simulink model "eVTOL_System"  (R2024b)
settings: Solver=FixedStepAuto  StartTime=0.0  StopTime=inf  RelTol=1e-3
undefined symbols (not defined in the file): airspeed, Battery, BCE12, BCE_Set_init, BMS_Controller_State, C, Cell10_P, Cell11_P, Cell12_P, Cell13_P, Cell14_P, Cell15_P, Cell16_P, Cell17_P, Cell18_P, Cell19_P, Cell1_N, Cell1_P, Cell20_P, Cell21_P, Cell22_P, Cell23_P, Cell24_P, Cell2_P, Cell3_P, Cell4_P, Cell5_P, Cell6_P, Cell7_P, Cell8_P, Cell9_P, Charging_State, CityMission, control, controlParams, ControlSampleTime, CriticalTiltAngle, currentFactor, CV_Gain, ddx, ddy, ddz, Device_01, Device_02, DiscIntNeverNeededParam, dx, dy, dz, Earth, env, F, F28379D_ADC_MaxCount, F28379D_ADC_Vmax, FixedWingMission, flightState, Foc_Ki_IxTcpu, Foc_Ki_S, Foc_Kp_I, Foc_Kp_S, fractalcoef ... (+68)
libraries: fl_lib x1115, nesl_utility x617, slrealtimeethercatlib x217, simulink x130, canmsglib x101, speedgoatlib_IO611_obsolete x91, slpidlib x49, mcbcontrolslib x44, slrealtimeutilitieslib x35, speedgoatlib_hdlCoder_IO3xx x31, dspstat3 x24, mcbpositiondecoderlib x12
(part 8 of 31)

== system eVTOL_System/Motor Drive/Controller/Controller_MIL/F28379D Firmware ==
  Ia_ADC : Inport
  Ib_ADC : Inport  Port=2
  IaOffset : Inport  Port=3
  IbOffset : Inport  Port=4
  QEP_Position_Count : Inport  Port=5
  QEP_Index_Latch : Inport  Port=6
  SpdCmdRPM : Inport  Port=7
  Kp_S : Inport  Port=8
  Ki_S : Inport  Port=9
  EnClosedLoop : Inport  Port=10
  EnablePWM : Inport  Port=11
  Kp_i : Inport  Port=12
  Ki_ixTcpu : Inport  Port=13
  Controller Algorithm : Subsystem
  Phase_Current_Rescaling : Subsystem
  Speed Conditioning : Subsystem
  ModWave : Outport
  PWM_Enable : Outport  Port=2
  Fbk_CAN : Outport  Port=3
  wires:
  SpdCmdRPM/1 -> Speed Conditioning/1(Spd[rpm])
  Ia_ADC/1 -> Phase_Current_Rescaling/1(Ia_ADC)
  IaOffset/1 -> Phase_Current_Rescaling/3(IaOffset)
  IbOffset/1 -> Phase_Current_Rescaling/4(IbOffset)
  QEP_Position_Count/1 -> Controller Algorithm/2(QEP_Position_Count)
  Controller Algorithm/1(ModWave) -> ModWave/1
  Phase_Current_Rescaling/1(Iab_meas_PU) -> Controller Algorithm/1(Ia_PU)  "Iab_fb_PU"
  Kp_S/1 -> Controller Algorithm/5(Kp_S)
  Controller Algorithm/2(PWM_Enable) -> PWM_Enable/1
  Ki_S/1 -> Controller Algorithm/6(Ki_S)
  QEP_Index_Latch/1 -> Controller Algorithm/3(QEP_Index_Latch)
  Ib_ADC/1 -> Phase_Current_Rescaling/2(Ib_ADC)
  EnClosedLoop/1 -> Controller Algorithm/7(EnClosedLoop)
  EnablePWM/1 -> Controller Algorithm/8(EnablePWM)
  Speed Conditioning/1(Spd[PU]) -> Controller Algorithm/4(SpdCmd)
  Controller Algorithm/3(fbk_CAN) -> Fbk_CAN/1
  Kp_i/1 -> Controller Algorithm/9(Kp_i)
  Ki_ixTcpu/1 -> Controller Algorithm/10(Ki_ixTcpu)

== system eVTOL_System/Motor Drive/Controller/Controller_MIL/IO334 DAC ==
  Iab : Inport
  Add : Sum
  Constant : Constant  Value=IO334_iDAC_bias
  Gain : Gain  Gain=IO334_iDAC_gain
  Gain1 : Gain  Gain=2.5/(2^15)
  IO334_DAC_embedded_GAIN : Gain  Gain=2^15/10
  Saturation : Saturate  UpperLimit=IO334_DAC_Vmax  LowerLimit=-IO334_DAC_Vmax
  Iab_IO334DAC : Outport
  wires:
  Iab/1 -> Gain/1
  Gain/1 -> Add/1
  Add/1 -> IO334_DAC_embedded_GAIN/1
  Constant/1 -> Add/2
  IO334_DAC_embedded_GAIN/1 -> Gain1/1
  Gain1/1 -> Saturation/1
  Saturation/1 -> Iab_IO334DAC/1

== system eVTOL_System/Motor Drive/Controller1/Controller_MIL/F28379D ADC ==
  Iab_IO334V : Inport
  Add Constant : Bias  Bias=Ia_offset  SaturateOnIntegerOverflow=off
  Add Constant1 : Bias  Bias=Ib_offset  SaturateOnIntegerOverflow=off
  Demux : Demux  Outputs=2
  Gain : Gain  Gain=2^12/F28379D_ADC_Vmax
  Ia_ADC : Outport
  Ib_ADC : Outport  Port=2
  wires:
  Iab_IO334V/1 -> Gain/1
  Gain/1 -> Demux/1
  Demux/1 -> Add Constant/1
  Demux/2 -> Add Constant1/1
  Add Constant/1 -> Ia_ADC/1
  Add Constant1/1 -> Ib_ADC/1

== system eVTOL_System/Motor Drive/Controller1/Controller_MIL/F28379D Firmware ==
  Ia_ADC : Inport
  Ib_ADC : Inport  Port=2
  IaOffset : Inport  Port=3
  IbOffset : Inport  Port=4
  QEP_Position_Count : Inport  Port=5
  QEP_Index_Latch : Inport  Port=6
  SpdCmdRPM : Inport  Port=7
  Kp_S : Inport  Port=8
  Ki_S : Inport  Port=9
  EnClosedLoop : Inport  Port=10
  EnablePWM : Inport  Port=11
  Kp_i : Inport  Port=12
  Ki_ixTcpu : Inport  Port=13
  Controller Algorithm : Subsystem
  Phase_Current_Rescaling : Subsystem
  Speed Conditioning : Subsystem
  ModWave : Outport
  PWM_Enable : Outport  Port=2
  Fbk_CAN : Outport  Port=3
  wires:
  SpdCmdRPM/1 -> Speed Conditioning/1(Spd[rpm])
  Ia_ADC/1 -> Phase_Current_Rescaling/1(Ia_ADC)
  IaOffset/1 -> Phase_Current_Rescaling/3(IaOffset)
  IbOffset/1 -> Phase_Current_Rescaling/4(IbOffset)
  QEP_Position_Count/1 -> Controller Algorithm/2(QEP_Position_Count)
  Controller Algorithm/1(ModWave) -> ModWave/1
  Phase_Current_Rescaling/1(Iab_meas_PU) -> Controller Algorithm/1(Ia_PU)  "Iab_fb_PU"
  Kp_S/1 -> Controller Algorithm/5(Kp_S)
  Controller Algorithm/2(PWM_Enable) -> PWM_Enable/1
  Ki_S/1 -> Controller Algorithm/6(Ki_S)
  QEP_Index_Latch/1 -> Controller Algorithm/3(QEP_Index_Latch)
  Ib_ADC/1 -> Phase_Current_Rescaling/2(Ib_ADC)
  EnClosedLoop/1 -> Controller Algorithm/7(EnClosedLoop)
  EnablePWM/1 -> Controller Algorithm/8(EnablePWM)
  Speed Conditioning/1(Spd[PU]) -> Controller Algorithm/4(SpdCmd)
  Controller Algorithm/3(fbk_CAN) -> Fbk_CAN/1
  Kp_i/1 -> Controller Algorithm/9(Kp_i)
  Ki_ixTcpu/1 -> Controller Algorithm/10(Ki_ixTcpu)

== system eVTOL_System/Motor Drive/Controller1/Controller_MIL/IO334 DAC ==
  Iab : Inport
  Add : Sum
  Constant : Constant  Value=IO334_iDAC_bias
  Gain : Gain  Gain=IO334_iDAC_gain
  Gain1 : Gain  Gain=2.5/(2^15)
  IO334_DAC_embedded_GAIN : Gain  Gain=2^15/10
  Saturation : Saturate  UpperLimit=IO334_DAC_Vmax  LowerLimit=-IO334_DAC_Vmax
  Iab_IO334DAC : Outport
  wires:
  Iab/1 -> Gain/1
  Gain/1 -> Add/1
  Add/1 -> IO334_DAC_embedded_GAIN/1
  Constant/1 -> Add/2
  IO334_DAC_embedded_GAIN/1 -> Gain1/1
  Gain1/1 -> Saturation/1
  Saturation/1 -> Iab_IO334DAC/1

== system eVTOL_System/Motor Drive/Controller2/Controller_MIL/F28379D ADC ==
  Iab_IO334V : Inport
  Add Constant : Bias  Bias=Ia_offset  SaturateOnIntegerOverflow=off
  Add Constant1 : Bias  Bias=Ib_offset  SaturateOnIntegerOverflow=off
  Demux : Demux  Outputs=2
  Gain : Gain  Gain=2^12/F28379D_ADC_Vmax
  Ia_ADC : Outport
  Ib_ADC : Outport  Port=2
  wires:
  Iab_IO334V/1 -> Gain/1
  Gain/1 -> Demux/1
  Demux/1 -> Add Constant/1
  Demux/2 -> Add Constant1/1
  Add Constant/1 -> Ia_ADC/1
  Add Constant1/1 -> Ib_ADC/1

== system eVTOL_System/Motor Drive/Controller2/Controller_MIL/F28379D Firmware ==
  Ia_ADC : Inport
  Ib_ADC : Inport  Port=2
  IaOffset : Inport  Port=3
  IbOffset : Inport  Port=4
  QEP_Position_Count : Inport  Port=5
  QEP_Index_Latch : Inport  Port=6
  SpdCmdRPM : Inport  Port=7
  Kp_S : Inport  Port=8
  Ki_S : Inport  Port=9
  EnClosedLoop : Inport  Port=10
  EnablePWM : Inport  Port=11
  Kp_i : Inport  Port=12
  Ki_ixTcpu : Inport  Port=13
  Controller Algorithm : Subsystem
  Phase_Current_Rescaling : Subsystem
  Speed Conditioning : Subsystem
  ModWave : Outport
  PWM_Enable : Outport  Port=2
  Fbk_CAN : Outport  Port=3
  wires:
  SpdCmdRPM/1 -> Speed Conditioning/1(Spd[rpm])
  Ia_ADC/1 -> Phase_Current_Rescaling/1(Ia_ADC)
  IaOffset/1 -> Phase_Current_Rescaling/3(IaOffset)
  IbOffset/1 -> Phase_Current_Rescaling/4(IbOffset)
  QEP_Position_Count/1 -> Controller Algorithm/2(QEP_Position_Count)
  Controller Algorithm/1(ModWave) -> ModWave/1
  Phase_Current_Rescaling/1(Iab_meas_PU) -> Controller Algorithm/1(Ia_PU)  "Iab_fb_PU"
  Kp_S/1 -> Controller Algorithm/5(Kp_S)
  Controller Algorithm/2(PWM_Enable) -> PWM_Enable/1
  Ki_S/1 -> Controller Algorithm/6(Ki_S)
  QEP_Index_Latch/1 -> Controller Algorithm/3(QEP_Index_Latch)
  Ib_ADC/1 -> Phase_Current_Rescaling/2(Ib_ADC)
  EnClosedLoop/1 -> Controller Algorithm/7(EnClosedLoop)
  EnablePWM/1 -> Controller Algorithm/8(EnablePWM)
  Speed Conditioning/1(Spd[PU]) -> Controller Algorithm/4(SpdCmd)
  Controller Algorithm/3(fbk_CAN) -> Fbk_CAN/1
  Kp_i/1 -> Controller Algorithm/9(Kp_i)
  Ki_ixTcpu/1 -> Controller Algorithm/10(Ki_ixTcpu)

== system eVTOL_System/Motor Drive/Controller2/Controller_MIL/IO334 DAC ==
  Iab : Inport
  Add : Sum
  Constant : Constant  Value=IO334_iDAC_bias
  Gain : Gain  Gain=IO334_iDAC_gain
  Gain1 : Gain  Gain=2.5/(2^15)
  IO334_DAC_embedded_GAIN : Gain  Gain=2^15/10
  Saturation : Saturate  UpperLimit=IO334_DAC_Vmax  LowerLimit=-IO334_DAC_Vmax
  Iab_IO334DAC : Outport
  wires:
  Iab/1 -> Gain/1
  Gain/1 -> Add/1
  Add/1 -> IO334_DAC_embedded_GAIN/1
  Constant/1 -> Add/2
  IO334_DAC_embedded_GAIN/1 -> Gain1/1
  Gain1/1 -> Saturation/1
  Saturation/1 -> Iab_IO334DAC/1

== system eVTOL_System/Motor Drive/Controller3/Controller_MIL/F28379D ADC ==
  Iab_IO334V : Inport
  Add Constant : Bias  Bias=Ia_offset  SaturateOnIntegerOverflow=off
  Add Constant1 : Bias  Bias=Ib_offset  SaturateOnIntegerOverflow=off
  Demux : Demux  Outputs=2
  Gain : Gain  Gain=2^12/F28379D_ADC_Vmax
  Ia_ADC : Outport
  Ib_ADC : Outport  Port=2
  wires:
  Iab_IO334V/1 -> Gain/1
  Gain/1 -> Demux/1
  Demux/1 -> Add Constant/1
  Demux/2 -> Add Constant1/1
  Add Constant/1 -> Ia_ADC/1
  Add Constant1/1 -> Ib_ADC/1

== system eVTOL_System/Motor Drive/Controller3/Controller_MIL/F28379D Firmware ==
  Ia_ADC : Inport
  Ib_ADC : Inport  Port=2
  IaOffset : Inport  Port=3
  IbOffset : Inport  Port=4
  QEP_Position_Count : Inport  Port=5
  QEP_Index_Latch : Inport  Port=6
  SpdCmdRPM : Inport  Port=7
  Kp_S : Inport  Port=8
  Ki_S : Inport  Port=9
  EnClosedLoop : Inport  Port=10
  EnablePWM : Inport  Port=11
  Kp_i : Inport  Port=12
  Ki_ixTcpu : Inport  Port=13
  Controller Algorithm : Subsystem
  Phase_Current_Rescaling : Subsystem
  Speed Conditioning : Subsystem
  ModWave : Outport
  PWM_Enable : Outport  Port=2
  Fbk_CAN : Outport  Port=3
  wires:
  SpdCmdRPM/1 -> Speed Conditioning/1(Spd[rpm])
  Ia_ADC/1 -> Phase_Current_Rescaling/1(Ia_ADC)
  IaOffset/1 -> Phase_Current_Rescaling/3(IaOffset)
  IbOffset/1 -> Phase_Current_Rescaling/4(IbOffset)
  QEP_Position_Count/1 -> Controller Algorithm/2(QEP_Position_Count)
  Controller Algorithm/1(ModWave) -> ModWave/1
  Phase_Current_Rescaling/1(Iab_meas_PU) -> Controller Algorithm/1(Ia_PU)  "Iab_fb_PU"
  Kp_S/1 -> Controller Algorithm/5(Kp_S)
  Controller Algorithm/2(PWM_Enable) -> PWM_Enable/1
  Ki_S/1 -> Controller Algorithm/6(Ki_S)
  QEP_Index_Latch/1 -> Controller Algorithm/3(QEP_Index_Latch)
  Ib_ADC/1 -> Phase_Current_Rescaling/2(Ib_ADC)
  EnClosedLoop/1 -> Controller Algorithm/7(EnClosedLoop)
  EnablePWM/1 -> Controller Algorithm/8(EnablePWM)
  Speed Conditioning/1(Spd[PU]) -> Controller Algorithm/4(SpdCmd)
  Controller Algorithm/3(fbk_CAN) -> Fbk_CAN/1
  Kp_i/1 -> Controller Algorithm/9(Kp_i)
  Ki_ixTcpu/1 -> Controller Algorithm/10(Ki_ixTcpu)

== system eVTOL_System/Motor Drive/Controller3/Controller_MIL/IO334 DAC ==
  Iab : Inport
  Add : Sum
  Constant : Constant  Value=IO334_iDAC_bias
  Gain : Gain  Gain=IO334_iDAC_gain
  Gain1 : Gain  Gain=2.5/(2^15)
  IO334_DAC_embedded_GAIN : Gain  Gain=2^15/10
  Saturation : Saturate  UpperLimit=IO334_DAC_Vmax  LowerLimit=-IO334_DAC_Vmax
  Iab_IO334DAC : Outport
  wires:
  Iab/1 -> Gain/1
  Gain/1 -> Add/1
  Add/1 -> IO334_DAC_embedded_GAIN/1
  Constant/1 -> Add/2
  IO334_DAC_embedded_GAIN/1 -> Gain1/1
  Gain1/1 -> Saturation/1
  Saturation/1 -> Iab_IO334DAC/1

== system eVTOL_System/Motor Drive/Three-Phase PMSM Drive/PMSM and average inverter/Encoder Simulation ==
  Theta_m : Inport
  Add1 : Sum  RndMeth=Simplest
  Data Type Conversion7 : DataTypeConversion  OutDataTypeStr=uint16  RndMeth=Simplest  SaturateOnIntegerOverflow=off
  "Get_PU " : Subsystem
  IndexOffset in PU : Constant  Value=0  OutDataTypeStr=single  SampleTime=-1
  Wrap : Subsystem
  pmsm.QEPSlits*4 : Gain  Gain=Maxon_Mile_Nslits*4  OutDataTypeStr=uint16  RndMeth=Simplest
  QEP_Position_Count : Outport
  wires:
  Add1/1 -> Wrap/1(in)
  Theta_m/1 -> "Get_PU "/1(rad)
  pmsm.QEPSlits*4/1 -> Data Type Conversion7/1  "Theta_e"
  Wrap/1(out) -> pmsm.QEPSlits*4/1  "theta_m(ideal)"
  IndexOffset in PU/1 -> Add1/2
  "Get_PU "/1(PU) -> Add1/1
  Data Type Conversion7/1 -> QEP_Position_Count/1

== system eVTOL_System/Motor Drive/Three-Phase PMSM Drive/PMSM and average inverter/Idc ==
  In1 : Inport
  Buffer : Buffer  N=154  OutputFrames=off
  Gain4 : Gain  Gain=1/10
  Gain7 : Gain  Gain=3/pi
  Gain8 : Gain  Gain=-1
  Square : Math  Operator=square
  Square Root : Sqrt
  Sum of Elements : Sum  Inputs=+
  Out1 : Outport
  wires:
  Square/1 -> Sum of Elements/1
  Square Root/1 -> Gain7/1  "Irms"
  Gain4/1 -> Square Root/1
  Gain7/1 -> Gain8/1  "Idc"
  In1/1 -> Buffer/1
  Sum of Elements/1 -> Gain4/1
  Buffer/1 -> Square/1
  Gain8/1 -> Out1/1

== system eVTOL_System/Motor Drive/Three-Phase PMSM Drive/PMSM and average inverter/Ideal Inverter ==
  V_DC : Inport
  Duty Cycle abc : Inport  Port=2
  Data Type Conversion : DataTypeConversion  OutDataTypeStr=single  SaturateOnIntegerOverflow=off  RndMeth=Floor
  Demux : Demux  Outputs=3
  Display1 : Display
  Display7 : Display
  Mux : Mux  Inputs=3
  Product : Product
  Product1 : Product
  Product2 : Product
  Vabc : Outport
  wires:
  V_DC/1 -> Display7/1, Product2/1, Product1/1, Product/1
  Demux/1 -> Product/2
  Duty Cycle abc/1 -> Data Type Conversion/1
  Mux/1 -> Vabc/1
  Data Type Conversion/1 -> Demux/1
  Demux/2 -> Product1/2
  Demux/3 -> Product2/2
  Product/1 -> Display1/1, Mux/1
  Product1/1 -> Mux/2
  Product2/1 -> Mux/3

== system eVTOL_System/Motor Drive/Three-Phase PMSM Drive/PMSM and average inverter/PMSM ==
  Config : Inport
  PhaseVolt abc : Inport  Port=2
  LdTrq / Spd : Inport  Port=3
  Constant : Constant  Value=0  OutDataTypeStr=boolean  SampleTime=-1
  PMSM HDL : mcbhdlplantlib/PMSM HDL  VariantControl=pmsmVariant==pmsmEnum.TorqueInput  Ts=Ts_CPU
      settings: LibrarySourceBlock=mcbhdllib/Electrical Systems/Motors/PMSM HDL
  Info : Outport
  PhaseCurr : Outport  Port=2
  Torque : Outport  Port=3
  RotorMechSpd : Outport  Port=4
  RotorElecAngle : Outport  Port=5
  wires:
  PMSM HDL/5 -> RotorElecAngle/1
  Config/1 -> PMSM HDL/1
  PMSM HDL/4 -> RotorMechSpd/1
  PMSM HDL/3 -> Torque/1
  PMSM HDL/2 -> PhaseCurr/1
  LdTrq / Spd/1 -> PMSM HDL/3
  PhaseVolt abc/1 -> PMSM HDL/2
  PMSM HDL/1 -> Info/1
  Constant/1 -> PMSM HDL/4

== system eVTOL_System/Motor Drive/Three-Phase PMSM Drive/PMSM and average inverter/Runtime to DC ==
  PWM_Runtime : Inport
  Demux : Demux  Outputs=15
  Mux : Mux  Inputs=3
  To Dc A1 : Subsystem
  To Dc A2 : Subsystem
  To Dc A3 : Subsystem
  Duty Cycle abc : Outport
  wires:
  PWM_Runtime/1 -> Demux/1  "PCIe_PWM_Runtime"
  Demux/2 -> To Dc A1/1(A_on)
  Demux/3 -> To Dc A1/2(A_off)
  Demux/7 -> To Dc A2/1(A_on)
  Demux/8 -> To Dc A2/2(A_off)
  Demux/12 -> To Dc A3/1(A_on)
  Demux/13 -> To Dc A3/2(A_off)
  To Dc A1/1(Dc) -> Mux/1
  To Dc A2/1(Dc) -> Mux/2
  To Dc A3/1(Dc) -> Mux/3
  Mux/1 -> Duty Cycle abc/1

== system eVTOL_System/Motor Drive/Three-Phase PMSM Drive/PMSM and inverter with switching dynamics/DAC Config ==
  I DAC bias : Constant  Value=IO334_iDAC_bias  OutDataTypeStr=single  SampleTime=Ts_UI
  I DAC gain : Constant  Value=IO334_iDAC_gain  OutDataTypeStr=single  SampleTime=Ts_UI
  Plant_Prequency : Constant  Value=1/ts_FPGA_mdl  SampleTime=Ts_UI
  Sig_frequ : Constant  Value=100000  VectorParams1D=off  SampleTime=Ts_UI
  Subsystem : Subsystem
  I_DAC_gain : Outport
  I_DAC_Current : Outport  Port=2
  DAC_reset : Outport  Port=3
  wires:
  Subsystem/1(DAC_reset) -> DAC_reset/1
  Plant_Prequency/1 -> Subsystem/1(Plant_frequency)
  Sig_frequ/1 -> Subsystem/2(SignalFrequency)
  I DAC gain/1 -> I_DAC_gain/1
  I DAC bias/1 -> I_DAC_Current/1

== system eVTOL_System/Motor Drive/Three-Phase PMSM Drive/PMSM and inverter with switching dynamics/Encoder Simulation ==
  Theta_m : Inport
  Add1 : Sum  RndMeth=Simplest
  Data Type Conversion7 : DataTypeConversion  OutDataTypeStr=uint16  RndMeth=Simplest  SaturateOnIntegerOverflow=off
  "Get_PU " : Subsystem
  IndexOffset in PU : Constant  Value=0  OutDataTypeStr=single  SampleTime=-1
  Wrap : Subsystem
  pmsm.QEPSlits*4 : Gain  Gain=Maxon_Mile_Nslits*4  OutDataTypeStr=uint16  RndMeth=Simplest
  QEP_Position_Count : Outport
  wires:
  Add1/1 -> Wrap/1(in)
  Theta_m/1 -> "Get_PU "/1(rad)
  pmsm.QEPSlits*4/1 -> Data Type Conversion7/1  "Theta_e"
  Wrap/1(out) -> pmsm.QEPSlits*4/1  "theta_m(ideal)"
  IndexOffset in PU/1 -> Add1/2
  "Get_PU "/1(PU) -> Add1/1
  Data Type Conversion7/1 -> QEP_Position_Count/1

== system eVTOL_System/Motor Drive/Three-Phase PMSM Drive/PMSM and inverter with switching dynamics/Idc ==
  In1 : Inport
  Buffer : Buffer  N=154  OutputFrames=off
  Gain4 : Gain  Gain=1/10
  Gain7 : Gain  Gain=3/pi
  Gain8 : Gain  Gain=-1
  Square : Math  Operator=square
  Square Root : Sqrt
  Sum of Elements : Sum  Inputs=+
  Out1 : Outport
  wires:
  Square/1 -> Sum of Elements/1
  Square Root/1 -> Gain7/1  "Irms"
  Gain4/1 -> Square Root/1
  Gain7/1 -> Gain8/1  "Idc"
  In1/1 -> Buffer/1
  Sum of Elements/1 -> Gain4/1
  Buffer/1 -> Square/1
  Gain8/1 -> Out1/1

== system eVTOL_System/Motor Drive/Three-Phase PMSM Drive/PMSM and inverter with switching dynamics/PMSM_3P2L_Inverter_Plant_TBR ==
  PCIe_RC_or_TTL : Inport
  PCIe_PWM_Config : Inport  Port=2
  PCIe_PWM_Runtime : Inport  Port=3
  PCIe_PWM_Enable : Inport  Port=4
  PCIe_Protocol : Inport  Port=5
  PCIe_V_dc : Inport  Port=6
  PCIe_Fault : Inport  Port=7
  PCIe_LdTrq/Spd : Inport  Port=8
  PCIe_Motor_Config : Inport  Port=9
  PCIe_Motor_Connection : Inport  Port=10
  PCIe_QAE_Config : Inport  Port=11
  PCIe_Resolver_Config : Inport  Port=12
  PCIe_Iabc_DAC_gain : Inport  Port=13
  PCIe_Iabc_DAC_bias : Inport  Port=14
  PCIe_DAC_reset : Inport  Port=15
  HIL_PWM_{0..5} (6 alike) : Constant  Value=0  OutDataTypeStr=boolean
  PMSM_3P2L_Inverter_Plant : Subsystem  mask(Speedgoat IO334-325k Interface Block){module_id=1, slot=-1, ts=-1, dacGain_1=10.0V, dacActiv_1=off, dacGain_2=2.5V, dacActiv_2=on, dacGain_3=2.5V, dacActiv_3=on, dacGain_4=2.5V, dacActiv_4=on, dacGain_5=2.5V, dacActiv_5=on, dacGain_6=10.0V, dacActiv_6=off, dacGain_7=2.5V, dacActiv_7=on, dacGain_8=10.0V, dacActiv_8=off, dacGain_9=10.0V, dacActiv_9=off, dacGain_10=10.0V, dacActiv_10=off, dacGain_11=10.0V, dacActiv_11=off, dacGain_12=10.0V, dacActiv_12=off, dacGain_13=10.0V, dacActiv_13=off, dacGain_14=10.0V, dacActiv_14=off, dacGain_15=10.0V, dacActiv_15=off, dacGain_16=10.0V, dacActiv_16=off, PullRPort0=pull-up 3.3V, VioPort0=3.3V, PullRPort1=pull-up 3.3V, VioPort1=3.3V, PullRPort2=pull-up 3.3V, VioPort2=3.3V, PullRPort3=pull-up 3.3V, VioPort3=3.3V, PullRPort4=pull-up 3.3V, VioPort4=3.3V, PullRPort5=pull-up 3.3V, VioPort5=3.3V, PullRPort6=pull-up 3.3V, VioPort6=3.3V, fpga_sync_mode=on, reset_mode=on, reset_mode_stop=on, FpgaFreq=200}
      mask prompts: module_id "FPGA Module Identifier:"; slot "PCI slot (-1: autosearch):"; ts "Sample time:"; dacGain_1 "DAC Ch 01 Range"; dacActiv_1 "Activ"; dacGain_2 "DAC Ch 02 Range"; dacActiv_2 "Activ"; dacGain_3 "DAC Ch 03 Range"; dacActiv_3 "Activ"; dacGain_4 "DAC Ch 04 Range"; dacActiv_4 "Activ"; dacGain_5 "DAC Ch 05 Range"; dacActiv_5 "Activ"; dacGain_6 "DAC Ch 06 Range"; dacActiv_6 "Activ"; dacGain_7 "DAC Ch 07 Range"; dacActiv_7 "Activ"; dacGain_8 "DAC Ch 08 Range"; dacActiv_8 "Activ"; dacGain_9 "DAC Ch 09 Range"; dacActiv_9 "Activ"; dacGain_10 "DAC Ch 10 Range"; dacActiv_10 "Activ"; dacGain_11 "DAC Ch 11 Range"; dacActiv_11 "Activ"; dacGain_12 "DAC Ch 12 Range"; dacActiv_12 "Activ"; dacGain_13 "DAC Ch 13 Range"; dacActiv_13 "Activ"; dacGain_14 "DAC Ch 14 Range"; dacActiv_14 "Activ"; dacGain_15 "DAC Ch 15 Range"; dacActiv_15 "Activ"; dacGain_16 "DAC Ch 16 Range"; dacActiv_16 "Activ"; PullRPort0 "pull resistor"; VioPort0 "I/O voltage"; PullRPort1 "pull resistor"; VioPort1 "I/O voltage"; PullRPort2 "pull resistor"; VioPort2 "I/O voltage"; PullRPort3 "pull resistor"; VioPort3 "I/O voltage"; PullRPort4 "pull resistor"; VioPort4 "I/O voltage"; PullRPort5 "pull resistor"; VioPort5 "I/O voltage"; PullRPort6 "pull resistor"; VioPort6 "I/O voltage"; fpga_sync_mode "Run FPGA only when target application runs"; reset_mode "Reset FPGA states on start"; reset_mode_stop "Reset FPGA states on stop"; FpgaFreq "FPGA Frequency [MHz]"
      mask help: Simulink Real-Time Interface Block for Speedgoat IO334-325k.
      mask init:
      | hdlslrt.backend.mfpgaparameters;
      | if sg.hdlc.utils.compareMatlabVersion('~=', 'R2024a')
      | 	sg.hdlc.warning(['The interface model that you are attempting to use was generated ',...
      | 		'in MATLAB R2024a and may not be compatible with the version you are currently using. ',...
      | 		'Attempting to use this interface model in a different MATLAB release can lead to ',...
      | 		'application crashes or other unpredictable behavior. ',...
      | 		'In order to avoid this and ensure stability and correct functionality, ',...
      | 		'we highly recommend regenerating the model with your current MATLAB release.']);
      | end
      mask Help: eval('speedgoatdoc_hdlc')
      mask TypeOptions dacGain_1: AD5547 Setup/dacGain_1
      mask TypeOptions dacActiv_1: AD5547 Setup/dacActiv_1
      mask TypeOptions dacGain_2: AD5547 Setup/dacGain_2
      mask TypeOptions dacActiv_2: AD5547 Setup/dacActiv_2
      mask TypeOptions dacGain_3: AD5547 Setup/dacGain_3
      mask TypeOptions dacActiv_3: AD5547 Setup/dacActiv_3
      mask TypeOptions dacGain_4: AD5547 Setup/dacGain_4
      mask TypeOptions dacActiv_4: AD5547 Setup/dacActiv_4
      mask TypeOptions dacGain_5: AD5547 Setup/dacGain_5
      mask TypeOptions dacActiv_5: AD5547 Setup/dacActiv_5
      mask TypeOptions dacGain_6: AD5547 Setup/dacGain_6
      mask TypeOptions dacActiv_6: AD5547 Setup/dacActiv_6
      mask TypeOptions dacGain_7: AD5547 Setup/dacGain_7
      mask TypeOptions dacActiv_7: AD5547 Setup/dacActiv_7
      mask TypeOptions dacGain_8: AD5547 Setup/dacGain_8
      mask TypeOptions dacActiv_8: AD5547 Setup/dacActiv_8
      mask TypeOptions dacGain_9: AD5547 Setup/dacGain_9
      mask TypeOptions dacActiv_9: AD5547 Setup/dacActiv_9
      mask TypeOptions dacGain_10: AD5547 Setup/dacGain_10
      mask TypeOptions dacActiv_10: AD5547 Setup/dacActiv_10
      mask TypeOptions dacGain_11: AD5547 Setup/dacGain_11
      mask TypeOptions dacActiv_11: AD5547 Setup/dacActiv_11
      mask TypeOptions dacGain_12: AD5547 Setup/dacGain_12
      mask TypeOptions dacActiv_12: AD5547 Setup/dacActiv_12
      mask TypeOptions dacGain_13: AD5547 Setup/dacGain_13
      mask TypeOptions dacActiv_13: AD5547 Setup/dacActiv_13
      mask TypeOptions dacGain_14: AD5547 Setup/dacGain_14
      mask TypeOptions dacActiv_14: AD5547 Setup/dacActiv_14
      mask TypeOptions dacGain_15: AD5547 Setup/dacGain_15
      mask TypeOptions dacActiv_15: AD5547 Setup/dacActiv_15
      mask TypeOptions dacGain_16: AD5547 Setup/dacGain_16
      mask TypeOptions dacActiv_16: AD5547 Setup/dacActiv_16
      mask TypeOptions PullRPort0: Port Settings -2x 0x00590000/PullRPort0
      mask Callback PullRPort0: sg_fpga_HDLCoder_io3xx_2x_m(2);
      mask TypeOptions VioPort0: Port Settings -2x 0x00590000/VioPort0
      mask Callback VioPort0: sg_fpga_HDLCoder_io3xx_2x_m(2);
      mask TypeOptions PullRPort1: Port Settings -2x 0x00590000/PullRPort1
      mask Callback PullRPort1: sg_fpga_HDLCoder_io3xx_2x_m(2);
      mask TypeOptions VioPort1: Port Settings -2x 0x00590000/VioPort1
      mask Callback VioPort1: sg_fpga_HDLCoder_io3xx_2x_m(2);
      mask TypeOptions PullRPort2: Port Settings -2x 0x00590000/PullRPort2
      mask Callback PullRPort2: sg_fpga_HDLCoder_io3xx_2x_m(2);
      mask TypeOptions VioPort2: Port Settings -2x 0x00590000/VioPort2
      mask Callback VioPort2: sg_fpga_HDLCoder_io3xx_2x_m(2);
      mask TypeOptions PullRPort3: Port Settings -2x 0x00590000/PullRPort3
      mask Callback PullRPort3: sg_fpga_HDLCoder_io3xx_2x_m(2);
      mask TypeOptions VioPort3: Port Settings -2x 0x00590000/VioPort3
      mask Callback VioPort3: sg_fpga_HDLCoder_io3xx_2x_m(2);
      mask TypeOptions PullRPort4: Port Settings -2x 0x00590000/PullRPort4
      mask Callback PullRPort4: sg_fpga_HDLCoder_io3xx_2x_m(2);
      mask TypeOptions VioPort4: Port Settings -2x 0x00590000/VioPort4
      mask Callback VioPort4: sg_fpga_HDLCoder_io3xx_2x_m(2);
      mask TypeOptions PullRPort5: Port Settings -2x 0x00590000/PullRPort5
      mask Callback PullRPort5: sg_fpga_HDLCoder_io3xx_2x_m(2);
      mask TypeOptions VioPort5: Port Settings -2x 0x00590000/VioPort5
      mask Callback VioPort5: sg_fpga_HDLCoder_io3xx_2x_m(2);
      mask TypeOptions PullRPort6: Port Settings -2x 0x00590000/PullRPort6
      mask Callback PullRPort6: sg_fpga_HDLCoder_io3xx_2x_m(2);
      mask TypeOptions VioPort6: Port Settings -2x 0x00590000/VioPort6
      mask Callback VioPort6: sg_fpga_HDLCoder_io3xx_2x_m(2);
      mask TypeOptions fpga_sync_mode: IO3xx Setup/fpga_sync_mode
      mask TypeOptions reset_mode: IO3xx Setup/reset_mode
      mask TypeOptions reset_mode_stop: IO3xx Setup/reset_mode_stop
      mask DialogControl DAC Prompt: DAC
      mask DialogControl dacGrp_1 Prompt: Ch 01 to 08
      mask DialogControl dacGrp_2 Prompt: Ch 09 to 16
      mask DialogControl IO33421 Prompt: IO334-21
      mask DialogControl port1 Prompt: Port 1
      mask DialogControl port2 Prompt: Port 2
      mask DialogControl port3 Prompt: Port 3
      mask DialogControl port4 Prompt: Port 4
      mask DialogControl port5 Prompt: Port 5
      mask DialogControl port6 Prompt: Port 6
      mask DialogControl port7 Prompt: Port 7
      mask Display:
      | SetupBlkPath = sghdlc.model.findSystem(gcb, 'LookUnderMasks', 'all', 'FollowLinks', 'on', 'regexp', 'on', 'Name', 'IO3(\d|x){2}\s+Setup' );
      | SetupBlkPath = SetupBlkPath{1};
      | TS = get_param(SetupBlkPath,'timestamp_mcs');
      | disp(sprintf('Speedgoat IO334-325k\nFPGA I/O Module\n\nTimestamp\n%s\n\nReference Design\nVersion 0.1\n\nMATLAB R2024a\n\nPCIe Link Width: X4\nTiming Severity: error\nRear Plugin: -21\nAurora Mode: None\nAurora Crc: true\nAurora Byteswap: true\nVerifier: off\nVerifier: JTAG\n', TS))
  Terminator{,1..10} (11 alike) : Terminator
  PCIe_Ia : Outport
  PCIe_Ib : Outport  Port=2
  PCIe_Ic : Outport  Port=3
  PCIe_Idc : Outport  Port=4
  PCIe_Motor_Spd : Outport  Port=5
  PCIe_Motor_Angle : Outport  Port=6
  PCIe_Motor_ElecAngle : Outport  Port=7
  PCIe_Motor_Trq : Outport  Port=8
  PCIe_Rsvl_excitation_pos : Outport  Port=9
  PCIe_Rsvl_excitation_neg : Outport  Port=10
  PCIe_Rsvl_sin_neg : Outport  Port=11
  PCIe_Rsvl_cos_neg : Outport  Port=12
  PCIe_Resolver_Out : Outport  Port=13
  wires:
  PCIe_RC_or_TTL/1 -> PMSM_3P2L_Inverter_Plant/1(PCIe_RC_or_TTL)
  PCIe_PWM_Config/1 -> PMSM_3P2L_Inverter_Plant/2(PCIe_PWM_Config)
  PCIe_PWM_Runtime/1 -> PMSM_3P2L_Inverter_Plant/3(PCIe_PWM_Runtime)
  PCIe_PWM_Enable/1 -> PMSM_3P2L_Inverter_Plant/4(PCIe_PWM_Enable)
  PCIe_Protocol/1 -> PMSM_3P2L_Inverter_Plant/5(PCIe_Protocol)
  PCIe_V_dc/1 -> PMSM_3P2L_Inverter_Plant/12(PCIe_V_dc)
  PCIe_Fault/1 -> PMSM_3P2L_Inverter_Plant/13(PCIe_Fault)
  PCIe_LdTrq/Spd/1 -> PMSM_3P2L_Inverter_Plant/14(PCIe_LdTrq/Spd)
  PCIe_Motor_Config/1 -> PMSM_3P2L_Inverter_Plant/15(PCIe_Motor_Config)
  PCIe_Motor_Connection/1 -> PMSM_3P2L_Inverter_Plant/16(PCIe_Motor_Connection)
  PCIe_QAE_Config/1 -> PMSM_3P2L_Inverter_Plant/17(PCIe_QAE_Config)
  PCIe_Resolver_Config/1 -> PMSM_3P2L_Inverter_Plant/18(PCIe_Resolver_Config)
  PCIe_DAC_reset/1 -> PMSM_3P2L_Inverter_Plant/21(PCIe_DAC_reset)
  PCIe_Iabc_DAC_bias/1 -> PMSM_3P2L_Inverter_Plant/20(PCIe_Iabc_DAC_bias)
  PCIe_Iabc_DAC_gain/1 -> PMSM_3P2L_Inverter_Plant/19(PCIe_Iabc_DAC_gain)
  PMSM_3P2L_Inverter_Plant/1(PCIe_Ia) -> PCIe_Ia/1
  PMSM_3P2L_Inverter_Plant/3(PCIe_Ic) -> PCIe_Ic/1
  PMSM_3P2L_Inverter_Plant/2(PCIe_Ib) -> PCIe_Ib/1
  PMSM_3P2L_Inverter_Plant/7(PCIe_Idc) -> PCIe_Idc/1
  PMSM_3P2L_Inverter_Plant/8(PCIe_Motor_Spd) -> PCIe_Motor_Spd/1
  PMSM_3P2L_Inverter_Plant/9(PCIe_Motor_Angle) -> PCIe_Motor_Angle/1
  PMSM_3P2L_Inverter_Plant/10(PCIe_Motor_ElecAngle) -> PCIe_Motor_ElecAngle/1
  PMSM_3P2L_Inverter_Plant/11(PCIe_Motor_Trq) -> PCIe_Motor_Trq/1
  PMSM_3P2L_Inverter_Plant/15(PCIe_Rsvl_excitation_pos) -> PCIe_Rsvl_excitation_pos/1
  PMSM_3P2L_Inverter_Plant/16(PCIe_Rsvl_excitation_neg) -> PCIe_Rsvl_excitation_neg/1
  PMSM_3P2L_Inverter_Plant/17(AO_5_Rsvl_sin_pos) -> Terminator10/1  "F28379D_A5"
  PMSM_3P2L_Inverter_Plant/18(PCIe_Rsvl_sin_neg) -> PCIe_Rsvl_sin_neg/1
  PMSM_3P2L_Inverter_Plant/20(PCIe_Rsvl_cos_neg) -> PCIe_Rsvl_cos_neg/1
  PMSM_3P2L_Inverter_Plant/21(PCIe_Resolver_Out) -> PCIe_Resolver_Out/1
  PMSM_3P2L_Inverter_Plant/22(TTL_32_Protocol) -> Terminator/1  "GPIO40"
  PMSM_3P2L_Inverter_Plant/23(TTL_24_AO_trigger_1_8) -> Terminator1/1
  PMSM_3P2L_Inverter_Plant/24(1_8_Null_AO_trigger) -> Terminator2/1
  PMSM_3P2L_Inverter_Plant/19(AO_7_Rsvl_cos_pos) -> Terminator3/1  "F28379D_C5"
  PMSM_3P2L_Inverter_Plant/14("TTL_50_QEP_A_I   ") -> Terminator6/1
  PMSM_3P2L_Inverter_Plant/12(TTL_48_QEP_A_A) -> Terminator4/1
  PMSM_3P2L_Inverter_Plant/13(TTL_49_QEP_A_B) -> Terminator5/1
  PMSM_3P2L_Inverter_Plant/6(AO_4_Ic) -> Terminator9/1  "F28379D_C4"
  PMSM_3P2L_Inverter_Plant/4(AO_2_Ia) -> Terminator7/1  "F28379D_A4"
  PMSM_3P2L_Inverter_Plant/5(AO_3_Ib) -> Terminator8/1  "F28379D_B4"
  HIL_PWM_0/1 -> PMSM_3P2L_Inverter_Plant/6(PWM1A TTL_0)
  HIL_PWM_1/1 -> PMSM_3P2L_Inverter_Plant/7(PWM1B TTL_1)
  HIL_PWM_2/1 -> PMSM_3P2L_Inverter_Plant/8(PWM2A TTL_2)
  HIL_PWM_3/1 -> PMSM_3P2L_Inverter_Plant/9(PWM2B TTL_3)
  HIL_PWM_4/1 -> PMSM_3P2L_Inverter_Plant/10(PWM3A TTL_4)
  HIL_PWM_5/1 -> PMSM_3P2L_Inverter_Plant/11(PWM3B TTL_5)

== system eVTOL_System/Motor Drive/Three-Phase PMSM Drive1/PMSM and average inverter/Encoder Simulation ==
  Theta_m : Inport
  Add1 : Sum  RndMeth=Simplest
  Data Type Conversion7 : DataTypeConversion  OutDataTypeStr=uint16  RndMeth=Simplest  SaturateOnIntegerOverflow=off
  "Get_PU " : Subsystem
  IndexOffset in PU : Constant  Value=0  OutDataTypeStr=single  SampleTime=-1
  Wrap : Subsystem
  pmsm.QEPSlits*4 : Gain  Gain=Maxon_Mile_Nslits*4  OutDataTypeStr=uint16  RndMeth=Simplest
  QEP_Position_Count : Outport
  wires:
  Add1/1 -> Wrap/1(in)
  Theta_m/1 -> "Get_PU "/1(rad)
  pmsm.QEPSlits*4/1 -> Data Type Conversion7/1  "Theta_e"
  Wrap/1(out) -> pmsm.QEPSlits*4/1  "theta_m(ideal)"
  IndexOffset in PU/1 -> Add1/2
  "Get_PU "/1(PU) -> Add1/1
  Data Type Conversion7/1 -> QEP_Position_Count/1

== system eVTOL_System/Motor Drive/Three-Phase PMSM Drive1/PMSM and average inverter/Idc ==
  In1 : Inport
  Buffer : Buffer  N=154  OutputFrames=off
  Gain1 : Gain  Gain=-1
  Gain4 : Gain  Gain=1/10
  Gain5 : Gain  Gain=1.414
  Gain6 : Gain  Gain=1/2
  Gain7 : Gain  Gain=3/pi
  Square : Math  Operator=square
  Square Root : Sqrt
  Sum of Elements : Sum  Inputs=+
  Terminator3 : Terminator
  Out1 : Outport
  wires:
  Gain7/1 -> Gain1/1  "Idc"
  Gain6/1 -> Terminator3/1  "Idc"
  Square Root/1 -> Gain7/1, Gain5/1  "Irms"
  Buffer/1 -> Square/1
  Sum of Elements/1 -> Gain4/1
  Gain4/1 -> Square Root/1
  Square/1 -> Sum of Elements/1
  Gain5/1 -> Gain6/1  "Ipeak"
  Gain1/1 -> Out1/1
  In1/1 -> Buffer/1

== system eVTOL_System/Motor Drive/Three-Phase PMSM Drive1/PMSM and average inverter/Ideal Inverter ==
  V_DC : Inport
  Duty Cycle abc : Inport  Port=2
  Data Type Conversion : DataTypeConversion  OutDataTypeStr=single  SaturateOnIntegerOverflow=off  RndMeth=Floor
  Demux : Demux  Outputs=3
  Mux : Mux  Inputs=3
  Product : Product
  Product1 : Product
  Product2 : Product
  Vabc : Outport
  wires:
  V_DC/1 -> Product2/1, Product1/1, Product/1
  Demux/1 -> Product/2
  Duty Cycle abc/1 -> Data Type Conversion/1
  Mux/1 -> Vabc/1
  Data Type Conversion/1 -> Demux/1
  Demux/2 -> Product1/2
  Demux/3 -> Product2/2
  Product/1 -> Mux/1
  Product1/1 -> Mux/2
  Product2/1 -> Mux/3

== system eVTOL_System/Motor Drive/Three-Phase PMSM Drive1/PMSM and average inverter/PMSM ==
  Config : Inport
  PhaseVolt abc : Inport  Port=2
  LdTrq / Spd : Inport  Port=3
  Constant : Constant  Value=0  OutDataTypeStr=boolean
  PMSM HDL : mcbhdlplantlib/PMSM HDL  VariantControl=pmsmVariant==pmsmEnum.TorqueInput  Ts=Ts_CPU
      settings: LibrarySourceBlock=mcbhdllib/Electrical Systems/Motors/PMSM HDL
  Info : Outport
  PhaseCurr : Outport  Port=2
  Torque : Outport  Port=3
  RotorMechSpd : Outport  Port=4
  RotorElecAngle : Outport  Port=5
  wires:
  PMSM HDL/5 -> RotorElecAngle/1
  Config/1 -> PMSM HDL/1
  PMSM HDL/4 -> RotorMechSpd/1
  PMSM HDL/3 -> Torque/1
  PMSM HDL/2 -> PhaseCurr/1
  LdTrq / Spd/1 -> PMSM HDL/3
  PhaseVolt abc/1 -> PMSM HDL/2
  PMSM HDL/1 -> Info/1
  Constant/1 -> PMSM HDL/4

== system eVTOL_System/Motor Drive/Three-Phase PMSM Drive1/PMSM and average inverter/Runtime to DC ==
  PWM_Runtime : Inport
  Demux : Demux  Outputs=15
  Mux : Mux  Inputs=3
  To Dc A1 : Subsystem
  To Dc A2 : Subsystem
  To Dc A3 : Subsystem
  Duty Cycle abc : Outport
  wires:
  PWM_Runtime/1 -> Demux/1  "PCIe_PWM_Runtime"
  Demux/2 -> To Dc A1/1(A_on)
  Demux/3 -> To Dc A1/2(A_off)
  Demux/7 -> To Dc A2/1(A_on)
  Demux/8 -> To Dc A2/2(A_off)
  Demux/12 -> To Dc A3/1(A_on)
  Demux/13 -> To Dc A3/2(A_off)
  To Dc A1/1(Dc) -> Mux/1
  To Dc A2/1(Dc) -> Mux/2
  To Dc A3/1(Dc) -> Mux/3
  Mux/1 -> Duty Cycle abc/1

== system eVTOL_System/Motor Drive/Three-Phase PMSM Drive2/PMSM and average inverter/Encoder Simulation ==
  Theta_m : Inport
  Add1 : Sum  RndMeth=Simplest
  Data Type Conversion7 : DataTypeConversion  OutDataTypeStr=uint16  RndMeth=Simplest  SaturateOnIntegerOverflow=off
  "Get_PU " : Subsystem
  IndexOffset in PU : Constant  Value=0  OutDataTypeStr=single  SampleTime=-1
  Wrap : Subsystem
  pmsm.QEPSlits*4 : Gain  Gain=Maxon_Mile_Nslits*4  OutDataTypeStr=uint16  RndMeth=Simplest
  QEP_Position_Count : Outport
  wires:
  Add1/1 -> Wrap/1(in)
  Theta_m/1 -> "Get_PU "/1(rad)
  pmsm.QEPSlits*4/1 -> Data Type Conversion7/1  "Theta_e"
  Wrap/1(out) -> pmsm.QEPSlits*4/1  "theta_m(ideal)"
  IndexOffset in PU/1 -> Add1/2
  "Get_PU "/1(PU) -> Add1/1
  Data Type Conversion7/1 -> QEP_Position_Count/1

== system eVTOL_System/Motor Drive/Three-Phase PMSM Drive2/PMSM and average inverter/Idc ==
  In1 : Inport
  Buffer : Buffer  N=154  OutputFrames=off
  Gain1 : Gain  Gain=-1
  Gain4 : Gain  Gain=1/10
  Gain5 : Gain  Gain=1.414
  Gain6 : Gain  Gain=1/2
  Gain7 : Gain  Gain=3/pi
  Square : Math  Operator=square
  Square Root : Sqrt
  Sum of Elements : Sum  Inputs=+
  Terminator3 : Terminator
  Out1 : Outport
  wires:
  Buffer/1 -> Square/1
  Gain5/1 -> Gain6/1  "Ipeak"
  Gain7/1 -> Gain1/1  "Idc"
  Square Root/1 -> Gain7/1, Gain5/1  "Irms"
  Gain4/1 -> Square Root/1
  Square/1 -> Sum of Elements/1
  Sum of Elements/1 -> Gain4/1
  Gain6/1 -> Terminator3/1  "Idc"
  In1/1 -> Buffer/1
  Gain1/1 -> Out1/1

== system eVTOL_System/Motor Drive/Three-Phase PMSM Drive2/PMSM and average inverter/Ideal Inverter ==
  V_DC : Inport
  Duty Cycle abc : Inport  Port=2
  Data Type Conversion : DataTypeConversion  OutDataTypeStr=single  SaturateOnIntegerOverflow=off  RndMeth=Floor
  Demux : Demux  Outputs=3
  Mux : Mux  Inputs=3
  Product : Product
  Product1 : Product
  Product2 : Product
  Vabc : Outport
  wires:
  V_DC/1 -> Product2/1, Product1/1, Product/1
  Demux/1 -> Product/2
  Duty Cycle abc/1 -> Data Type Conversion/1
  Mux/1 -> Vabc/1
  Data Type Conversion/1 -> Demux/1
  Demux/2 -> Product1/2
  Demux/3 -> Product2/2
  Product/1 -> Mux/1
  Product1/1 -> Mux/2
  Product2/1 -> Mux/3

== system eVTOL_System/Motor Drive/Three-Phase PMSM Drive2/PMSM and average inverter/PMSM ==
  Config : Inport
  PhaseVolt abc : Inport  Port=2
  LdTrq / Spd : Inport  Port=3
  Constant : Constant  Value=0  OutDataTypeStr=boolean
  PMSM HDL : mcbhdlplantlib/PMSM HDL  VariantControl=pmsmVariant==pmsmEnum.TorqueInput  Ts=Ts_CPU
      settings: LibrarySourceBlock=mcbhdllib/Electrical Systems/Motors/PMSM HDL
  Info : Outport
  PhaseCurr : Outport  Port=2
  Torque : Outport  Port=3
  RotorMechSpd : Outport  Port=4
  RotorElecAngle : Outport  Port=5
  wires:
  PMSM HDL/5 -> RotorElecAngle/1
  Config/1 -> PMSM HDL/1
  PMSM HDL/4 -> RotorMechSpd/1
  PMSM HDL/3 -> Torque/1
  PMSM HDL/2 -> PhaseCurr/1
  LdTrq / Spd/1 -> PMSM HDL/3
  PhaseVolt abc/1 -> PMSM HDL/2
  PMSM HDL/1 -> Info/1
  Constant/1 -> PMSM HDL/4

== system eVTOL_System/Motor Drive/Three-Phase PMSM Drive2/PMSM and average inverter/Runtime to DC ==
  PWM_Runtime : Inport
  Demux : Demux  Outputs=15
  Mux : Mux  Inputs=3
  To Dc A1 : Subsystem
  To Dc A2 : Subsystem
  To Dc A3 : Subsystem
  Duty Cycle abc : Outport
  wires:
  PWM_Runtime/1 -> Demux/1  "PCIe_PWM_Runtime"
  Demux/2 -> To Dc A1/1(A_on)
  Demux/3 -> To Dc A1/2(A_off)
  Demux/7 -> To Dc A2/1(A_on)
  Demux/8 -> To Dc A2/2(A_off)
  Demux/12 -> To Dc A3/1(A_on)
  Demux/13 -> To Dc A3/2(A_off)
  To Dc A1/1(Dc) -> Mux/1
  To Dc A2/1(Dc) -> Mux/2
  To Dc A3/1(Dc) -> Mux/3
  Mux/1 -> Duty Cycle abc/1

== system eVTOL_System/Motor Drive/Three-Phase PMSM Drive3/PMSM and average inverter/Encoder Simulation ==
  Theta_m : Inport
  Add1 : Sum  RndMeth=Simplest
  Data Type Conversion7 : DataTypeConversion  OutDataTypeStr=uint16  RndMeth=Simplest  SaturateOnIntegerOverflow=off
  "Get_PU " : Subsystem
  IndexOffset in PU : Constant  Value=0  OutDataTypeStr=single  SampleTime=-1
  Wrap : Subsystem
  pmsm.QEPSlits*4 : Gain  Gain=Maxon_Mile_Nslits*4  OutDataTypeStr=uint16  RndMeth=Simplest
  QEP_Position_Count : Outport
  wires:
  Add1/1 -> Wrap/1(in)
  Theta_m/1 -> "Get_PU "/1(rad)
  pmsm.QEPSlits*4/1 -> Data Type Conversion7/1  "Theta_e"
  Wrap/1(out) -> pmsm.QEPSlits*4/1  "theta_m(ideal)"
  IndexOffset in PU/1 -> Add1/2
  "Get_PU "/1(PU) -> Add1/1
  Data Type Conversion7/1 -> QEP_Position_Count/1

== system eVTOL_System/Motor Drive/Three-Phase PMSM Drive3/PMSM and average inverter/Idc ==
  In1 : Inport
  Buffer : Buffer  N=154  OutputFrames=off
  Gain1 : Gain  Gain=-1
  Gain4 : Gain  Gain=1/10
  Gain5 : Gain  Gain=1.414
  Gain6 : Gain  Gain=1/2
  Gain7 : Gain  Gain=3/pi
  Square : Math  Operator=square
  Square Root : Sqrt
  Sum of Elements : Sum  Inputs=+
  Terminator3 : Terminator
  Out1 : Outport
  wires:
  Gain7/1 -> Gain1/1  "Idc"
  Gain6/1 -> Terminator3/1  "Idc"
  Buffer/1 -> Square/1
  Square Root/1 -> Gain7/1, Gain5/1  "Irms"
  Square/1 -> Sum of Elements/1
  Sum of Elements/1 -> Gain4/1
  Gain4/1 -> Square Root/1
  Gain5/1 -> Gain6/1  "Ipeak"
  Gain1/1 -> Out1/1
  In1/1 -> Buffer/1

== system eVTOL_System/Motor Drive/Three-Phase PMSM Drive3/PMSM and average inverter/Ideal Inverter ==
  V_DC : Inport
  Duty Cycle abc : Inport  Port=2
  Data Type Conversion : DataTypeConversion  OutDataTypeStr=single  SaturateOnIntegerOverflow=off  RndMeth=Floor
  Demux : Demux  Outputs=3
  Mux : Mux  Inputs=3
  Product : Product
  Product1 : Product
  Product2 : Product
  Vabc : Outport
  wires:
  V_DC/1 -> Product2/1, Product1/1, Product/1
  Demux/1 -> Product/2
  Duty Cycle abc/1 -> Data Type Conversion/1
  Mux/1 -> Vabc/1
  Data Type Conversion/1 -> Demux/1
  Demux/2 -> Product1/2
  Demux/3 -> Product2/2
  Product/1 -> Mux/1
  Product1/1 -> Mux/2
  Product2/1 -> Mux/3

== system eVTOL_System/Motor Drive/Three-Phase PMSM Drive3/PMSM and average inverter/PMSM ==
  Config : Inport
  PhaseVolt abc : Inport  Port=2
  LdTrq / Spd : Inport  Port=3
  Constant : Constant  Value=0  OutDataTypeStr=boolean
  PMSM HDL : mcbhdlplantlib/PMSM HDL  VariantControl=pmsmVariant==pmsmEnum.TorqueInput  Ts=Ts_CPU
      settings: LibrarySourceBlock=mcbhdllib/Electrical Systems/Motors/PMSM HDL
  Info : Outport
  PhaseCurr : Outport  Port=2
  Torque : Outport  Port=3
  RotorMechSpd : Outport  Port=4
  RotorElecAngle : Outport  Port=5
  wires:
  PMSM HDL/5 -> RotorElecAngle/1
  Config/1 -> PMSM HDL/1
  PMSM HDL/4 -> RotorMechSpd/1
  PMSM HDL/3 -> Torque/1
  PMSM HDL/2 -> PhaseCurr/1
  LdTrq / Spd/1 -> PMSM HDL/3
  PhaseVolt abc/1 -> PMSM HDL/2
  PMSM HDL/1 -> Info/1
  Constant/1 -> PMSM HDL/4

== system eVTOL_System/Motor Drive/Three-Phase PMSM Drive3/PMSM and average inverter/Runtime to DC ==
  PWM_Runtime : Inport
  Demux : Demux  Outputs=15
  Mux : Mux  Inputs=3
  To Dc A1 : Subsystem
  To Dc A2 : Subsystem
  To Dc A3 : Subsystem
  Duty Cycle abc : Outport
  wires:
  PWM_Runtime/1 -> Demux/1  "PCIe_PWM_Runtime"
  Demux/2 -> To Dc A1/1(A_on)
  Demux/3 -> To Dc A1/2(A_off)
  Demux/7 -> To Dc A2/1(A_on)
  Demux/8 -> To Dc A2/2(A_off)
  Demux/12 -> To Dc A3/1(A_on)
  Demux/13 -> To Dc A3/2(A_off)
  To Dc A1/1(Dc) -> Mux/1
  To Dc A2/1(Dc) -> Mux/2
  To Dc A3/1(Dc) -> Mux/3
  Mux/1 -> Duty Cycle abc/1

== system eVTOL_System/Visualization/Photorealistic/PhotorealisticHIL/Prepare UAV Data ==
  UAVState : Inport
  Bus Selector1 : BusSelector  OutputSignals=x,y,z,yaw,pitch,roll
  Gain{,1..3} (4 alike) : Gain  Gain=-1
  Mux : Mux  Inputs=3
  Mux1 : Mux  Inputs=3
  Translation : Outport
  Rotation : Outport  Port=2
  wires:
  UAVState/1 -> Bus Selector1/1
  Mux/1 -> Translation/1
  Mux1/1 -> Rotation/1  "EulerZYX"
  Bus Selector1/4 -> Gain3/1  "<yaw>"
  Bus Selector1/5 -> Gain2/1  "<pitch>"
  Bus Selector1/6 -> Mux1/3  "<roll>"
  Bus Selector1/3 -> Gain/1  "<z>"
  Bus Selector1/2 -> Gain1/1  "<y>"
  Bus Selector1/1 -> Mux/1  "<x>"
  Gain/1 -> Mux/3
  Gain1/1 -> Mux/2
  Gain2/1 -> Mux1/2
  Gain3/1 -> Mux1/1

== system eVTOL_System/Visualization/Photorealistic/PhotorealisticMIL/Prepare UAV Data ==
  UAVState : Inport
  Bus Selector1 : BusSelector  OutputSignals=x,y,z,yaw,pitch,roll
  Gain{,1..3} (4 alike) : Gain  Gain=-1
  Mux : Mux  Inputs=3
  Mux1 : Mux  Inputs=3
  Translation : Outport
  Rotation : Outport  Port=2
  wires:
  UAVState/1 -> Bus Selector1/1
  Mux/1 -> Translation/1
  Mux1/1 -> Rotation/1  "EulerZYX"
  Bus Selector1/4 -> Gain3/1  "<yaw>"
  Bus Selector1/5 -> Gain2/1  "<pitch>"
  Bus Selector1/6 -> Mux1/3  "<roll>"
  Bus Selector1/3 -> Gain/1  "<z>"
  Bus Selector1/2 -> Gain1/1  "<y>"
  Bus Selector1/1 -> Mux/1  "<x>"
  Gain/1 -> Mux/3
  Gain1/1 -> Mux/2
  Gain2/1 -> Mux1/2
  Gain3/1 -> Mux1/1

== system eVTOL_System/Visualization/Visualization/VisualizationMIL/Subsystem ==
  <Xe> : Inport
  <q> : Inport  Port=2
  RotorA : Inport  Port=3
  RotorB : Inport  Port=4
  Constant : Constant  Value=0
  Constant1 : Constant  Value=0
  Gain : Gain  Gain=0
  Gain1 : Gain  Gain=-1
  Gain2 : Gain  Gain=-1
  MATLAB System : MATLABSystem  System=exampleHelperTiltRotorAnimator  SampleTime=0.05
      mask Type: exampleHelperTiltRotorAnimator
      mask Display:
      | disp('exampleHelperTiltRotorAnimator');
      | port_label('input',1,'position');
      | port_label('input',2,'orientation');
      | port_label('input',3,'rotorAngles');
  Mux : Mux
  Reshape : Reshape  OutputDimensionality=Customize  OutputDimensions=[1,4]
  Reshape1 : Reshape  OutputDimensionality=Customize  OutputDimensions=[1,4]
  Reshape2 : Reshape  OutputDimensionality=Customize  OutputDimensions=[1,3]
  wires:
  Gain1/1 -> Mux/1
  Constant1/1 -> Mux/4
  Gain2/1 -> Mux/2
  Reshape1/1 -> MATLAB System/3
  Mux/1 -> Reshape1/1
  RotorA/1 -> Gain1/1
  <Xe>/1 -> Gain/1
  Constant/1 -> Mux/3
  RotorB/1 -> Gain2/1
  <q>/1 -> Reshape/1
  Reshape2/1 -> MATLAB System/1
  Reshape/1 -> MATLAB System/2
  Gain/1 -> Reshape2/1

== system eVTOL_System/Battery System/BMS/HIL/Cell Monitoring Unit/Balancing_Circuit3 ==
  Bal_Cmd_Controller : Inport
  38-Cell : Subsystem  VariantControl=Ns_Module == 12
  Cells : PMIOPort  Side=Left
  Balancing_Currents : Outport
  wires:
  Bal_Cmd_Controller/1 -> 38-Cell/1(Bal_Cmd_Controller)
  38-Cell/1(Balancing_Currents) -> Balancing_Currents/1
  connections:
  Cells/RConn1 -- 38-Cell/LConn1

== system eVTOL_System/Battery System/BMS/HIL/Cell Monitoring Unit/Balancing_Circuit4 ==
  Bal_Cmd_Controller : Inport
  38-Cell : Subsystem  VariantControl=Ns_Module == 12
  Cells : PMIOPort  Side=Left
  Balancing_Currents : Outport
  wires:
  Bal_Cmd_Controller/1 -> 38-Cell/1(Bal_Cmd_Controller)
  38-Cell/1(Balancing_Currents) -> Balancing_Currents/1
  connections:
  Cells/RConn1 -- 38-Cell/LConn1

== system eVTOL_System/Battery System/BMS/HIL/Cell Monitoring Unit/CMU1 ==
  Bal_Cmd_Controller : Inport
  38-Cell : Subsystem  VariantControl=Ns_Module == 12
  Cells : PMIOPort  Side=Left
  Balancing_Currents : Outport
  wires:
  Bal_Cmd_Controller/1 -> 38-Cell/1(Bal_Cmd_Controller)
  38-Cell/1(Balancing_Currents) -> Balancing_Currents/1
  connections:
  Cells/RConn1 -- 38-Cell/LConn1

== system eVTOL_System/Battery System/BMS/HIL/Cell Monitoring Unit/CMU2 ==
  Bal_Cmd_Controller : Inport
  38-Cell : Subsystem  VariantControl=Ns_Module == 12
  Cells : PMIOPort  Side=Left
  Balancing_Currents : Outport
  wires:
  Bal_Cmd_Controller/1 -> 38-Cell/1(Bal_Cmd_Controller)
  38-Cell/1(Balancing_Currents) -> Balancing_Currents/1
  connections:
  Cells/RConn1 -- 38-Cell/LConn1

== system eVTOL_System/Battery System/BMS/HIL/Controller_100Cells/PLANT-Rx ==
  CAN Read : speedgoatlib_IO611_obsolete/CAN/CAN Read  id=1  sampleTime=-1  portSelection=2  messageType=CAN  BusOutput=off  protl=IO611  ptIdx=1  isFDMod=1
      settings: SourceProductName=IO611
  Data Type Conversion{,1..3} (4 alike) : DataTypeConversion  OutDataTypeStr=single  SaturateOnIntegerOverflow=off  RndMeth=Floor
  Messages : Subsystem
  While Iterator : WhileIterator  MaxIters=-1  WhileBlockType=do-while
  BMS_Faults : Outport
  Charging_State : Outport  Port=2
  BMS_State : Outport  Port=3
  SOC : Outport  Port=4
  Discharge_Current_Limit : Outport  Port=5
  Charge_Current_Limit : Outport  Port=6
  Charge_Current_Req : Outport  Port=7
  Bal_Cmd_76Cells : Outport  Port=8
  wires:
  CAN Read/2 -> Messages/6(ID_0x204), Messages/5(ID_0x203), Messages/4(ID_0x502), Messages/3(ID_0x501), Messages/2(ID_0x202), Messages/1(ID_0x201)
  CAN Read/1 -> While Iterator/1
  Messages/1(Discharge_Current_Limit) -> Data Type Conversion/1
  Messages/7(Charging_State) -> Charging_State/1
  Messages/2(Charge_Current_Limit) -> Data Type Conversion1/1
  Messages/3(Charge_Current_Req) -> Data Type Conversion2/1
  Messages/4(SOC) -> Data Type Conversion3/1
  Messages/6(BMS_State) -> BMS_State/1
  Data Type Conversion/1 -> Discharge_Current_Limit/1
  Data Type Conversion1/1 -> Charge_Current_Limit/1
  Data Type Conversion2/1 -> Charge_Current_Req/1
  Data Type Conversion3/1 -> SOC/1
  Messages/5(BMS_Faults) -> BMS_Faults/1
  Messages/8(Bal_Cmd_76Cells) -> Bal_Cmd_76Cells/1

== system eVTOL_System/Battery System/BMS/HIL/Controller_100Cells/PLANT-Tx ==
  to_Controller : Inport
  to_Controller_SRE : Inport  Port=2
  24-Cell : Subsystem  VariantControl=Ns_Module == 12
  wires:
  to_Controller/1 -> 24-Cell/1(to_Controller)
  to_Controller_SRE/1 -> 24-Cell/2(to_Controller_SRE)

== system eVTOL_System/Battery System/BMS/HIL/Controller_76Cells/BMS State Machine ==
  Discharge_Current_Limit : Inport
  Charge_Current_Limit : Inport  Port=2
  State_Request : Inport  Port=3  OutDataTypeStr=Enum: SRE
  Sensor_Values : Inport  Port=4
  Fault_Reset_Enable : Inport  Port=5
  Bus Selector : BusSelector  OutputSignals=Cell_Voltages,Pack_Voltage2,Cell_Temperatures,Pack_Current
  Data Type Conversion : DataTypeConversion  OutDataTypeStr=boolean  SaturateOnIntegerOverflow=off  RndMeth=Floor
  Selector1 : Subsystem
  Selector3 : Subsystem
  State_Machine : Stateflow chart  TreatAsAtomicUnit=on  VariantControl=(default)
  Charge_Current_Req : Outport  OutMin=-100  OutMax=100  OutDataTypeStr=single  VectorParamsAs1DForOutWhenUnconnected=off
  Faults : Outport  Port=2  OutDataTypeStr=Bus: Faults  VectorParamsAs1DForOutWhenUnconnected=off  BusOutputAsStruct=on
  Charging_State : Outport  Port=3
  BMS_State : Outport  Port=4  OutDataTypeStr=Enum: BMS_Controller_State  VectorParamsAs1DForOutWhenUnconnected=off
  wires:
  State_Machine/2(Fault_out) -> Faults/1  "Faults"
  Bus Selector/1 -> Selector3/1(In1)  "<Cell_Voltages>"
  State_Machine/1(ChargeCurrentReq) -> Charge_Current_Req/1  "Charge_Current_Req"
  State_Request/1 -> State_Machine/3(State_Request)
  Discharge_Current_Limit/1 -> State_Machine/1(DischargeCurrentLimit)
  Charge_Current_Limit/1 -> State_Machine/2(ChargeCurrentLimit)
  Bus Selector/3 -> Selector1/1(In1)  "<Cell_Temperatures>"
  Bus Selector/2 -> State_Machine/5(Pack_Voltage)  "<Pack_Voltage2>"
  Bus Selector/4 -> State_Machine/7(Pack_Current)  "<Pack_Current>"
  Sensor_Values/1 -> Bus Selector/1
  Fault_Reset_Enable/1 -> Data Type Conversion/1
  Data Type Conversion/1 -> State_Machine/8(Fault_Reset_Enable)
  State_Machine/3(ChargeModeReq) -> Charging_State/1  "Charging_State"
  State_Machine/4(BMS_State) -> BMS_State/1  "BMS_State"
  Selector3/1(Out1) -> State_Machine/4(Cell_Voltages)
  Selector1/1(Out1) -> State_Machine/6(Cell_Temperatures)

== system eVTOL_System/Battery System/BMS/HIL/Controller_76Cells/Balancing Logic ==
  BMS_State : Inport  OutDataTypeStr=Enum: BMS_Controller_State  PortDimensions=1
  Sensor_Values : Inport  Port=2
  Balancing : Stateflow chart  TreatAsAtomicUnit=on  VariantControl=(default)
  Bus Selector1 : BusSelector  OutputSignals=Cell_Voltages
  Selector1 : Subsystem
  Bal_Cmd1 : Outport  OutDataTypeStr=boolean  PortDimensions=[1,76]  VectorParamsAs1DForOutWhenUnconnected=off
  wires:
  Bus Selector1/1 -> Selector1/1(In1)  "<Cell_Voltages>"
  Sensor_Values/1 -> Bus Selector1/1
  BMS_State/1 -> Balancing/1(BMS_State)
  Selector1/1(Out1) -> Balancing/2(CellVoltages)
  Balancing/1(Bal_Cmd1) -> Bal_Cmd1/1  "Bal_Cmd1"
